simulink model "SimulinkRoboticHand"  (R2025a)
settings: Solver=VariableStepAuto  StartTime=0.0  StopTime=2  RelTol=1e-3
undefined symbols (not defined in the file): Kd, Kp, q_contatto
libraries: roblocks x15
settings Model: Creator=gbluc  LastModifiedBy=gbluc

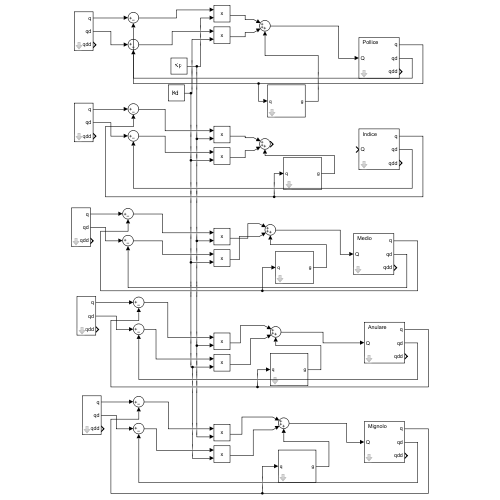
[thumbnail: Simulink's stored preview of the top-level diagram]
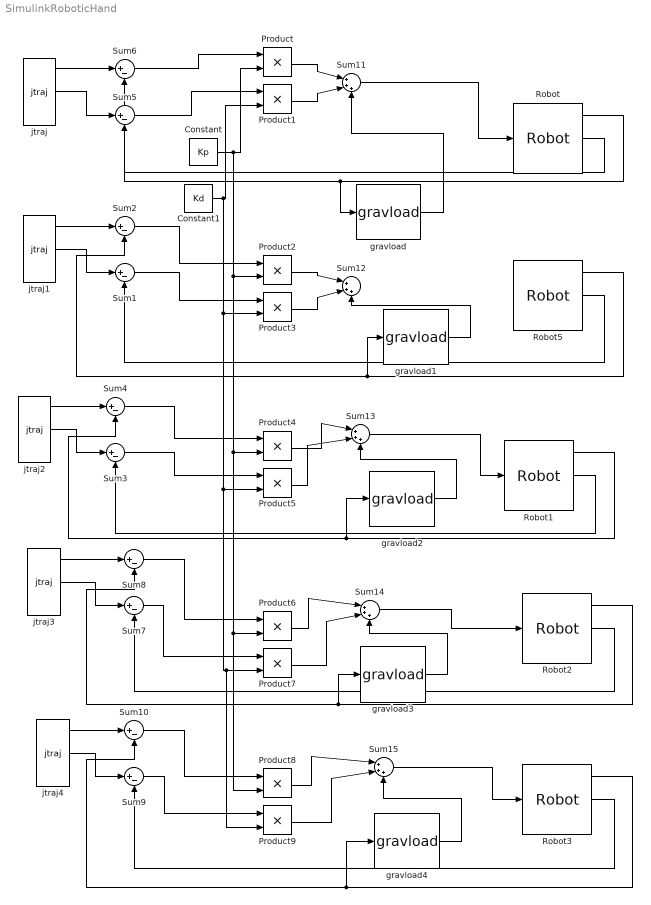
== system SimulinkRoboticHand ==
  Constant : Constant  Value=Kp
  Constant1 : Constant  Value=Kd
  Product{,1..9} (10 alike) : Product
  Robot : roblocks/Arm/Robot  robot=robot  q0=[0 0 0]
  Robot1 : roblocks/Arm/Robot  robot=medio  q0=[0 0 0]
  Robot2 : roblocks/Arm/Robot  robot=anulare  q0=[0 0 0]
  Robot3 : roblocks/Arm/Robot  robot=mignolo  q0=[0 0 0]
  Robot5 : roblocks/Arm/Robot  robot=indice  q0=[0 0 0]
  Sum{1..10} (10 alike) : Sum  Inputs=|+-
  Sum{11..15} (5 alike) : Sum  Inputs=|+++
  gravload : roblocks/Arm/gravload  robot=pollice
  gravload1 : roblocks/Arm/gravload  robot=indice
  gravload2 : roblocks/Arm/gravload  robot=medio
  gravload3 : roblocks/Arm/gravload  robot=anulare
  gravload4 : roblocks/Arm/gravload  robot=mignolo
  jtraj : roblocks/Toolbox/jtraj  q0=[0 0 0]  qf=q_contatto{5}  tmax=1.5  ts=0.001
  jtraj1 : roblocks/Toolbox/jtraj  q0=[0 0 0]  qf=q_contatto{1}  tmax=1.5  ts=0.001
  jtraj2 : roblocks/Toolbox/jtraj  q0=[0 0 0]  qf=q_contatto{2}  tmax=1.5  ts=0.001
  jtraj3 : roblocks/Toolbox/jtraj  q0=[0 0 0]  qf=q_contatto{3}  tmax=1.5  ts=0.001
  jtraj4 : roblocks/Toolbox/jtraj  q0=[0 0 0]  qf=q_contatto{4}  tmax=1.5  ts=0.001
  wires:
  jtraj/1 -> Sum6/1
  jtraj/2 -> Sum5/1
  Robot/1 -> gravload/1, Sum6/2
  Robot/2 -> Sum5/2
  jtraj1/2 -> Sum1/1
  Robot5/2 -> Sum1/2
  jtraj1/1 -> Sum2/1
  Robot5/1 -> gravload1/1, Sum2/2
  jtraj2/2 -> Sum3/1
  Robot1/2 -> Sum3/2
  jtraj2/1 -> Sum4/1
  Robot1/1 -> gravload2/1, Sum4/2
  jtraj3/2 -> Sum7/1
  Robot2/2 -> Sum7/2
  jtraj3/1 -> Sum8/1
  Robot2/1 -> gravload3/1, Sum8/2
  jtraj4/2 -> Sum9/1
  Robot3/2 -> Sum9/2
  jtraj4/1 -> Sum10/1
  Robot3/1 -> gravload4/1, Sum10/2
  Constant/1 -> Product8/2, Product6/2, Product4/2, Product2/2, Product/2
  Constant1/1 -> Product9/2, Product7/2, Product5/2, Product3/2, Product1/2
  Sum6/1 -> Product/1
  Sum5/1 -> Product1/1
  Sum2/1 -> Product2/1
  Sum1/1 -> Product3/1
  Sum4/1 -> Product4/1
  Sum3/1 -> Product5/1
  Sum8/1 -> Product6/1
  Sum7/1 -> Product7/1
  Sum10/1 -> Product8/1
  Sum9/1 -> Product9/1
  Product/1 -> Sum11/1
  Product1/1 -> Sum11/2
  gravload/1 -> Sum11/3
  Sum11/1 -> Robot/1
  Product2/1 -> Sum12/1
  Product3/1 -> Sum12/2
  gravload1/1 -> Sum12/3
  Product4/1 -> Sum13/1
  Product5/1 -> Sum13/2
  gravload2/1 -> Sum13/3
  Product9/1 -> Sum15/2
  Product8/1 -> Sum15/1
  gravload4/1 -> Sum15/3
  Sum15/1 -> Robot3/1
  gravload3/1 -> Sum14/3
  Product7/1 -> Sum14/2
  Product6/1 -> Sum14/1
  Sum13/1 -> Robot1/1
  Sum14/1 -> Robot2/1
